simulink library "commsync"  (Simulink 5.0)
libraries: commutil x6
settings Model: Creator=mikem  LastModifiedBy=mmclerno

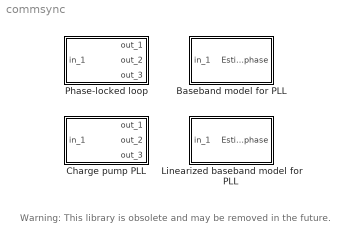
== system commsync ==
  note: Warning:  This library is obsolete and may be
      | removed in the future.
  Baseband model for PLL : Subsystem  mask(Baseband PLL model){Fn=[3.0002,  0, 40002], Fd=[1, 67.46, 2270.9, 40002], Ac=1, G=2}
      mask prompts: Fn "Lowpass filter numerator:"; Fd "Lowpass filter denominator:"; Ac "Oscillation amplitude:"; G "Gain at the output:"
      mask help: Output the phase shifting of the input signal from the oscillation frequency.
      mask init:
      | pi2=2*pi;Kc=Ac/2;
      mask Help: this block is used to detect the phase shifting of the input signal. The input to this block is an oscillation signal with possible phase shifting. The block detects the phase shifting value using the PLL technique. Design the lowpass filter to pass the phase changing signal and to eliminate the oscillation signal.
      mask Display: disp('Baseband\nPLL')
  Charge pump PLL : Subsystem  mask(Charge pump PLL){Fn=[3.0002,  0, 40002], Fd=[1, 67.46, 2270.9, 40002], Fc=100/2/pi, Ph=pi, Ac=1, G=3}
      mask prompts: Fn "Lowpass filter numerator:"; Fd "Lowpass filter Denominator:"; Fc "Oscillation frequency (Hz):"; Ph "Oscillation Phase (rad):"; Ac "Oscillation Amplitude:"; G "Gain at the output:"
      mask help: Output the phase shifting signal at 1st port; the detected phase error at 2nd port; VOC output at 3rd port.
      mask init:
      | Cu=1;
      mask Help: This block uses a digital charge pump to detect the phase shifting from the oscillation signal. The first output is the detected phase shift. The second output is the detected phase error output from phase detector. The third output is the matching signal for the input. Note a 180 degree phase difference between the input signal and the matching signal.
      mask Display: disp('Charge\npump\nPLL')
  Linearized baseband model for PLL : Subsystem  mask(Linearized baseband PLL model){Fn=[3.0002,  0, 40002], Fd=[1, 67.46, 2270.9, 40002], Ac=1, G=2}
      mask prompts: Fn "Lowpass filter numerator:"; Fd "Lowpass filter denominator:"; Ac "Oscillation amplitude:"; G "Gain at the output:"
      mask help: Output the phase shifting of the input signal from the oscillation frequency.
      mask init:
      | pi2=2*pi;Kc=Ac/2;
      mask Help: This block detects the phase shifting of the input signal. The input to this block is an oscillation signal with possible phase shifting. The block detects the phase shifting value using PLL technique. Design the lowpass filter to pass the phase changing signal and to eliminate the oscillation signal.
      mask Display: disp('Linearized\nbaseband\nPLL')
  Phase-locked loop : Subsystem  mask(Simple form PLL){Fn=[3.0002,  0, 40002], Fd=[1, 67.46, 2270.9, 40002], Fc=100/2/pi, Ph=pi/2, Ac=1, G=2}
      mask prompts: Fn "Lowpass filter numerator:"; Fd "Lowpass filter denominator:"; Fc "Oscillation frequency:"; Ph "Oscillation Phase:"; Ac "Oscillation Amplitude:"; G "Gain at the output:"
      mask help: Output the phase shifting signal at 1st port; the detected phase error at 2nd port; VOC output at 3rd port.
      mask Help: This block detects the phase shifting of the input signal. This block uses a multiplier phase detector. The first output is the detected phase shift. The second output is the detected phase error output from phase detector. The third output is the matching signal for the input. Note a 180 degree phase difference between the input signal and the matching signal.
      mask Display: disp('PLL')

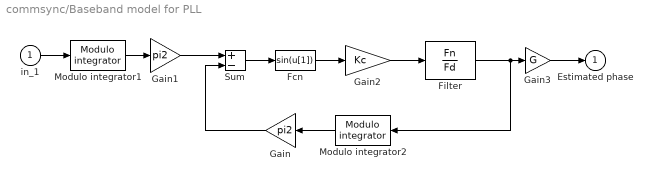
== system commsync/Baseband model for PLL ==
  in_1 : Inport
  Fcn : Fcn
  Filter : TransferFcn  Numerator=Fn  Denominator=Fd
  Gain : Gain  Orientation=left  Gain=pi2  SaturateOnIntegerOverflow=on
  Gain1 : Gain  Gain=pi2  SaturateOnIntegerOverflow=on
  Gain2 : Gain  Gain=Kc  SaturateOnIntegerOverflow=on
  Gain3 : Gain  Gain=G  SaturateOnIntegerOverflow=on
  Modulo integrator1 : commutil/Modulo integrator  modu=1  init=0
  Modulo integrator2 : commutil/Modulo integrator  Orientation=left  modu=1  init=0
  Sum : Sum  Inputs=+-  SaturateOnIntegerOverflow=on  InputSameDT=on
  Estimated phase : Outport  InitialOutput=0
  wires:
  in_1/1 -> Modulo integrator1/1
  Fcn/1 -> Gain2/1
  Sum/1 -> Fcn/1
  Filter/1 -> Modulo integrator2/1, Gain3/1
  Modulo integrator2/1 -> Gain/1
  Modulo integrator1/1 -> Gain1/1
  Gain3/1 -> Estimated phase/1
  Gain2/1 -> Filter/1
  Gain1/1 -> Sum/1
  Gain/1 -> Sum/2

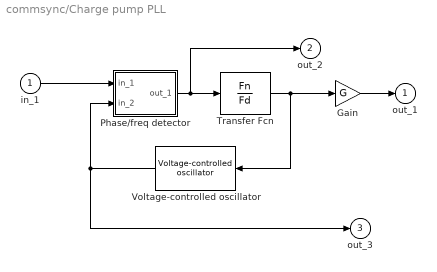
== system commsync/Charge pump PLL ==
  in_1 : Inport
  Gain : Gain  Gain=G  SaturateOnIntegerOverflow=on
  Phase/freq detector : Subsystem  mask(Phase Detector){@1=-sqrt(eps), @2=Cu}
      mask prompts: @1 "Cross zero line threshold:"; @2 "Charge pump current:"
      mask help: Phase detector:
      mask init:
      | Thre=@1;Cu=@2;lo=[0 0;0 1;1 0;1 0;0 1;0 1;0 0;0 0;1 0;0 0;1 0;0 0;1 0;0 0;0 0;0 0];
      mask Display: disp('Phase\nfrequency\ndetector')
  Transfer Fcn : TransferFcn  Numerator=Fn  Denominator=Fd
  Voltage-controlled oscillator : commutil/Voltage-controlled oscillator  Orientation=left  Ac=Ac  Fc=Fc  Kc=1  Ph=Ph
  out_1 : Outport  InitialOutput=0
  out_2 : Outport  Port=2  InitialOutput=0
  out_3 : Outport  Port=3  InitialOutput=0
  wires:
  Transfer Fcn/1 -> Gain/1, Voltage-controlled oscillator/1
  Gain/1 -> out_1/1
  in_1/1 -> Phase/freq detector/1(in_1)
  Voltage-controlled oscillator/1 -> Phase/freq detector/2(in_2), out_3/1
  Phase/freq detector/1(out_1) -> Transfer Fcn/1, out_2/1

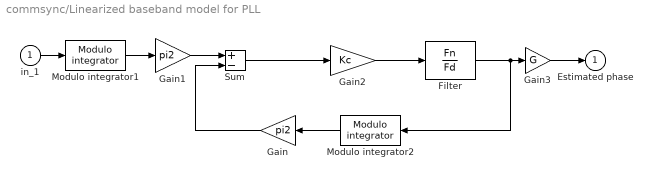
== system commsync/Linearized baseband model for PLL ==
  in_1 : Inport
  Filter : TransferFcn  Numerator=Fn  Denominator=Fd
  Gain : Gain  Orientation=left  Gain=pi2  SaturateOnIntegerOverflow=on
  Gain1 : Gain  Gain=pi2  SaturateOnIntegerOverflow=on
  Gain2 : Gain  Gain=Kc  SaturateOnIntegerOverflow=on
  Gain3 : Gain  Gain=G  SaturateOnIntegerOverflow=on
  Modulo integrator1 : commutil/Modulo integrator  modu=1  init=0
  Modulo integrator2 : commutil/Modulo integrator  Orientation=left  modu=1  init=0
  Sum : Sum  Inputs=+-  SaturateOnIntegerOverflow=on  InputSameDT=on
  Estimated phase : Outport  InitialOutput=0
  wires:
  in_1/1 -> Modulo integrator1/1
  Gain/1 -> Sum/2
  Gain1/1 -> Sum/1
  Gain2/1 -> Filter/1
  Gain3/1 -> Estimated phase/1
  Modulo integrator1/1 -> Gain1/1
  Modulo integrator2/1 -> Gain/1
  Filter/1 -> Modulo integrator2/1, Gain3/1
  Sum/1 -> Gain2/1

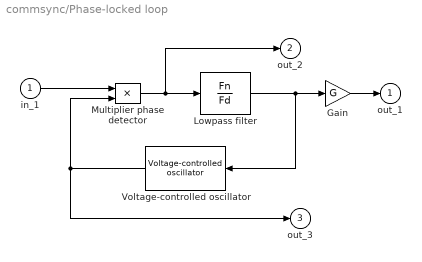
== system commsync/Phase-locked loop ==
  in_1 : Inport
  Gain : Gain  Gain=G  SaturateOnIntegerOverflow=on
  Lowpass filter : TransferFcn  Numerator=Fn  Denominator=Fd
  Multiplier phase detector : Product  SaturateOnIntegerOverflow=on  InputSameDT=on
  Voltage-controlled oscillator : commutil/Voltage-controlled oscillator  Orientation=left  Ac=Ac  Fc=Fc  Kc=1  Ph=Ph
  out_1 : Outport  InitialOutput=0
  out_2 : Outport  Port=2  InitialOutput=0
  out_3 : Outport  Port=3  InitialOutput=0
  wires:
  Gain/1 -> out_1/1
  Lowpass filter/1 -> Voltage-controlled oscillator/1, Gain/1
  in_1/1 -> Multiplier phase detector/1
  Multiplier phase detector/1 -> Lowpass filter/1, out_2/1
  Voltage-controlled oscillator/1 -> Multiplier phase detector/2, out_3/1

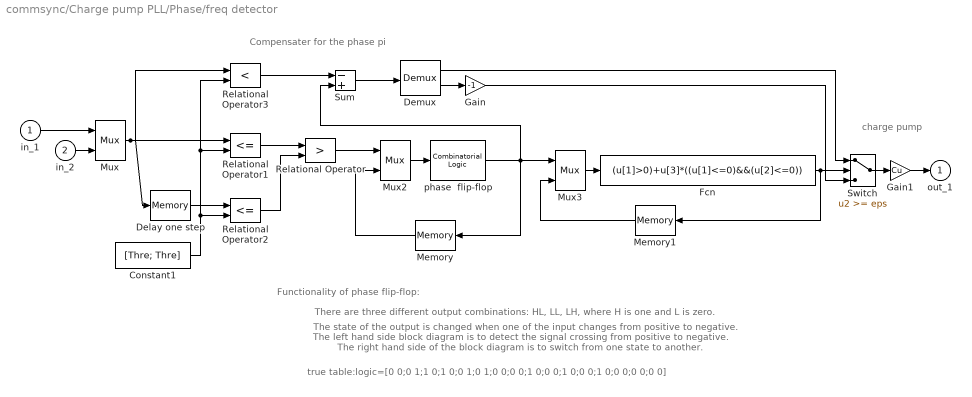
== system commsync/Charge pump PLL/Phase/freq detector ==
  note: Compensater for the phase pi
  note: charge pump
  note: Functionality of phase flip-flop:
  note: The left hand side block diagram is to detect the signal crossing from positive to negative.
      | The right hand side of the block diagram is to switch from one state to another.
  note: The state of the output is changed when one of the input changes from positive to negative.
  note: There are three different output combinations: HL, LL, LH, where H is one and L is zero.
  note: true table:logic=[0 0;0 1;1 0;1 0;0 1;0 1;0 0;0 0;1 0;0 0;1 0;0 0;1 0;0 0;0 0;0 0]
  in_1 : Inport
  in_2 : Inport  Port=2
  Constant1 : Constant  Value=[Thre; Thre]
  Delay one step : Memory
  Demux : Demux  Outputs=2
  Fcn : Fcn  Expr=(u[1]>0)+u[3]*((u[1]<=0)&&(u[2]<=0))
  Gain : Gain  Gain=-1  SaturateOnIntegerOverflow=on
  Gain1 : Gain  Gain=Cu  SaturateOnIntegerOverflow=on
  Memory : Memory  Orientation=left
  Memory1 : Memory  Orientation=left
  Mux : Mux  Inputs=2
  Mux2 : Mux  Inputs=[2 2]
  Mux3 : Mux  Inputs=[2 1]
  Relational Operator : RelationalOperator  Operator=>  InputSameDT=on
  Relational Operator1 : RelationalOperator  Operator=<=  InputSameDT=on
  Relational Operator2 : RelationalOperator  Operator=<=  InputSameDT=on
  Relational Operator3 : RelationalOperator  Operator=<  InputSameDT=on
  Sum : Sum  Inputs=-+  SaturateOnIntegerOverflow=on  InputSameDT=on
  Switch : Switch  Threshold=eps  SaturateOnIntegerOverflow=on  InputSameDT=on
  phase  flip-flop : CombinatorialLogic  TruthTable=lo
  out_1 : Outport  InitialOutput=0
  wires:
  Switch/1 -> Gain1/1
  Demux/1 -> Switch/1
  Gain/1 -> Switch/3
  Demux/2 -> Gain/1
  Sum/1 -> Demux/1
  phase  flip-flop/1 -> Memory/1, Mux3/1, Sum/2
  Relational Operator3/1 -> Sum/1
  Fcn/1 -> Switch/2, Memory1/1
  Mux3/1 -> Fcn/1
  Memory1/1 -> Mux3/2
  Constant1/1 -> Relational Operator2/2, Relational Operator3/2, Relational Operator1/2
  Mux/1 -> Relational Operator3/1, Delay one step/1, Relational Operator1/1
  Memory/1 -> Mux2/2
  Gain1/1 -> out_1/1
  Relational Operator2/1 -> Relational Operator/2
  Relational Operator1/1 -> Relational Operator/1
  Delay one step/1 -> Relational Operator2/1
  Mux2/1 -> phase  flip-flop/1
  Relational Operator/1 -> Mux2/1
  in_2/1 -> Mux/2
  in_1/1 -> Mux/1
